simulink model "8Bit_Processor"  (R2019b)
settings: Solver=FixedStepDiscrete  StartTime=0.0  StopTime=10.0  RelTol=1e-3
libraries: hdlsllib x127, simulink_extras x9
(part 2 of 4)

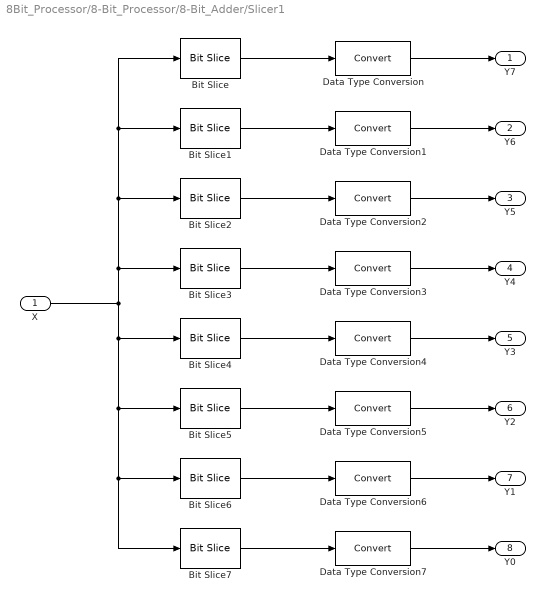
== system 8Bit_Processor/8-Bit_Processor/8-Bit_Adder/Slicer1 ==
  X : Inport  OutDataTypeStr=uint8  SampleTime=1
  Bit Slice : hdlsllib/Logic and Bit Operations/Bit Slice  lidx=7  ridx=7
      settings: SourceProductName=Simulink  SourceProductBaseCode=SL
  Bit Slice1 : hdlsllib/Logic and Bit Operations/Bit Slice  lidx=6  ridx=6
      settings: SourceProductName=Simulink  SourceProductBaseCode=SL
  Bit Slice2 : hdlsllib/Logic and Bit Operations/Bit Slice  lidx=5  ridx=5
      settings: SourceProductName=Simulink  SourceProductBaseCode=SL
  Bit Slice3 : hdlsllib/Logic and Bit Operations/Bit Slice  lidx=4  ridx=4
      settings: SourceProductName=Simulink  SourceProductBaseCode=SL
  Bit Slice4 : hdlsllib/Logic and Bit Operations/Bit Slice  lidx=3  ridx=3
      settings: SourceProductName=Simulink  SourceProductBaseCode=SL
  Bit Slice5 : hdlsllib/Logic and Bit Operations/Bit Slice  lidx=2  ridx=2
      settings: SourceProductName=Simulink  SourceProductBaseCode=SL
  Bit Slice6 : hdlsllib/Logic and Bit Operations/Bit Slice  lidx=1  ridx=1
      settings: SourceProductName=Simulink  SourceProductBaseCode=SL
  Bit Slice7 : hdlsllib/Logic and Bit Operations/Bit Slice  lidx=0  ridx=0
      settings: SourceProductName=Simulink  SourceProductBaseCode=SL
  Data Type Conversion{,1..7} (8 alike) : DataTypeConversion
  Y7 : Outport
  Y6 : Outport  Port=2
  Y5 : Outport  Port=3
  Y4 : Outport  Port=4
  Y3 : Outport  Port=5
  Y2 : Outport  Port=6
  Y1 : Outport  Port=7
  Y0 : Outport  Port=8
  wires:
  Bit Slice6/1 -> Data Type Conversion6/1
  X/1 -> Bit Slice3/1, Bit Slice2/1, Bit Slice1/1, Bit Slice/1, Bit Slice4/1, Bit Slice5/1, Bit Slice6/1, Bit Slice7/1
  Bit Slice/1 -> Data Type Conversion/1
  Bit Slice7/1 -> Data Type Conversion7/1
  Bit Slice4/1 -> Data Type Conversion4/1
  Bit Slice1/1 -> Data Type Conversion1/1
  Bit Slice3/1 -> Data Type Conversion3/1
  Data Type Conversion1/1 -> Y6/1
  Data Type Conversion7/1 -> Y0/1
  Data Type Conversion5/1 -> Y2/1
  Data Type Conversion3/1 -> Y4/1
  Data Type Conversion4/1 -> Y3/1
  Bit Slice2/1 -> Data Type Conversion2/1
  Bit Slice5/1 -> Data Type Conversion5/1
  Data Type Conversion6/1 -> Y1/1
  Data Type Conversion/1 -> Y7/1
  Data Type Conversion2/1 -> Y5/1

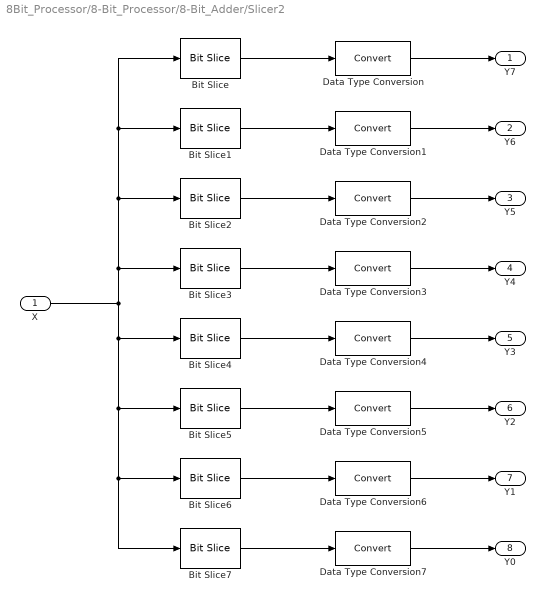
== system 8Bit_Processor/8-Bit_Processor/8-Bit_Adder/Slicer2 ==
  X : Inport  OutDataTypeStr=uint8  SampleTime=1
  Bit Slice : hdlsllib/Logic and Bit Operations/Bit Slice  lidx=7  ridx=7
      settings: SourceProductName=Simulink  SourceProductBaseCode=SL
  Bit Slice1 : hdlsllib/Logic and Bit Operations/Bit Slice  lidx=6  ridx=6
      settings: SourceProductName=Simulink  SourceProductBaseCode=SL
  Bit Slice2 : hdlsllib/Logic and Bit Operations/Bit Slice  lidx=5  ridx=5
      settings: SourceProductName=Simulink  SourceProductBaseCode=SL
  Bit Slice3 : hdlsllib/Logic and Bit Operations/Bit Slice  lidx=4  ridx=4
      settings: SourceProductName=Simulink  SourceProductBaseCode=SL
  Bit Slice4 : hdlsllib/Logic and Bit Operations/Bit Slice  lidx=3  ridx=3
      settings: SourceProductName=Simulink  SourceProductBaseCode=SL
  Bit Slice5 : hdlsllib/Logic and Bit Operations/Bit Slice  lidx=2  ridx=2
      settings: SourceProductName=Simulink  SourceProductBaseCode=SL
  Bit Slice6 : hdlsllib/Logic and Bit Operations/Bit Slice  lidx=1  ridx=1
      settings: SourceProductName=Simulink  SourceProductBaseCode=SL
  Bit Slice7 : hdlsllib/Logic and Bit Operations/Bit Slice  lidx=0  ridx=0
      settings: SourceProductName=Simulink  SourceProductBaseCode=SL
  Data Type Conversion{,1..7} (8 alike) : DataTypeConversion
  Y7 : Outport
  Y6 : Outport  Port=2
  Y5 : Outport  Port=3
  Y4 : Outport  Port=4
  Y3 : Outport  Port=5
  Y2 : Outport  Port=6
  Y1 : Outport  Port=7
  Y0 : Outport  Port=8
  wires:
  Bit Slice6/1 -> Data Type Conversion6/1
  X/1 -> Bit Slice3/1, Bit Slice2/1, Bit Slice1/1, Bit Slice/1, Bit Slice4/1, Bit Slice5/1, Bit Slice6/1, Bit Slice7/1
  Bit Slice/1 -> Data Type Conversion/1
  Bit Slice7/1 -> Data Type Conversion7/1
  Bit Slice4/1 -> Data Type Conversion4/1
  Bit Slice1/1 -> Data Type Conversion1/1
  Bit Slice3/1 -> Data Type Conversion3/1
  Data Type Conversion1/1 -> Y6/1
  Data Type Conversion7/1 -> Y0/1
  Data Type Conversion5/1 -> Y2/1
  Data Type Conversion3/1 -> Y4/1
  Data Type Conversion4/1 -> Y3/1
  Bit Slice2/1 -> Data Type Conversion2/1
  Bit Slice5/1 -> Data Type Conversion5/1
  Data Type Conversion6/1 -> Y1/1
  Data Type Conversion/1 -> Y7/1
  Data Type Conversion2/1 -> Y5/1

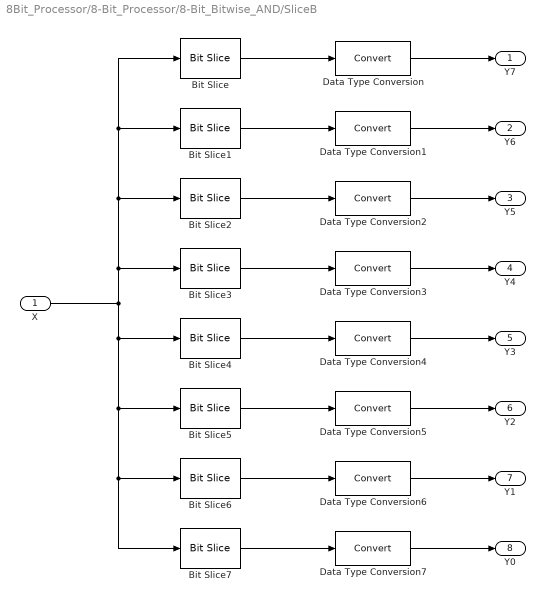
== system 8Bit_Processor/8-Bit_Processor/8-Bit_Bitwise_AND/SliceB ==
  X : Inport  OutDataTypeStr=uint8  SampleTime=1
  Bit Slice : hdlsllib/Logic and Bit Operations/Bit Slice  lidx=7  ridx=7
      settings: SourceProductName=Simulink  SourceProductBaseCode=SL
  Bit Slice1 : hdlsllib/Logic and Bit Operations/Bit Slice  lidx=6  ridx=6
      settings: SourceProductName=Simulink  SourceProductBaseCode=SL
  Bit Slice2 : hdlsllib/Logic and Bit Operations/Bit Slice  lidx=5  ridx=5
      settings: SourceProductName=Simulink  SourceProductBaseCode=SL
  Bit Slice3 : hdlsllib/Logic and Bit Operations/Bit Slice  lidx=4  ridx=4
      settings: SourceProductName=Simulink  SourceProductBaseCode=SL
  Bit Slice4 : hdlsllib/Logic and Bit Operations/Bit Slice  lidx=3  ridx=3
      settings: SourceProductName=Simulink  SourceProductBaseCode=SL
  Bit Slice5 : hdlsllib/Logic and Bit Operations/Bit Slice  lidx=2  ridx=2
      settings: SourceProductName=Simulink  SourceProductBaseCode=SL
  Bit Slice6 : hdlsllib/Logic and Bit Operations/Bit Slice  lidx=1  ridx=1
      settings: SourceProductName=Simulink  SourceProductBaseCode=SL
  Bit Slice7 : hdlsllib/Logic and Bit Operations/Bit Slice  lidx=0  ridx=0
      settings: SourceProductName=Simulink  SourceProductBaseCode=SL
  Data Type Conversion{,1..7} (8 alike) : DataTypeConversion
  Y7 : Outport
  Y6 : Outport  Port=2
  Y5 : Outport  Port=3
  Y4 : Outport  Port=4
  Y3 : Outport  Port=5
  Y2 : Outport  Port=6
  Y1 : Outport  Port=7
  Y0 : Outport  Port=8
  wires:
  Bit Slice6/1 -> Data Type Conversion6/1
  X/1 -> Bit Slice3/1, Bit Slice2/1, Bit Slice1/1, Bit Slice/1, Bit Slice4/1, Bit Slice5/1, Bit Slice6/1, Bit Slice7/1
  Bit Slice/1 -> Data Type Conversion/1
  Bit Slice7/1 -> Data Type Conversion7/1
  Bit Slice4/1 -> Data Type Conversion4/1
  Bit Slice1/1 -> Data Type Conversion1/1
  Bit Slice3/1 -> Data Type Conversion3/1
  Data Type Conversion1/1 -> Y6/1
  Data Type Conversion7/1 -> Y0/1
  Data Type Conversion5/1 -> Y2/1
  Data Type Conversion3/1 -> Y4/1
  Data Type Conversion4/1 -> Y3/1
  Bit Slice2/1 -> Data Type Conversion2/1
  Bit Slice5/1 -> Data Type Conversion5/1
  Data Type Conversion6/1 -> Y1/1
  Data Type Conversion/1 -> Y7/1
  Data Type Conversion2/1 -> Y5/1

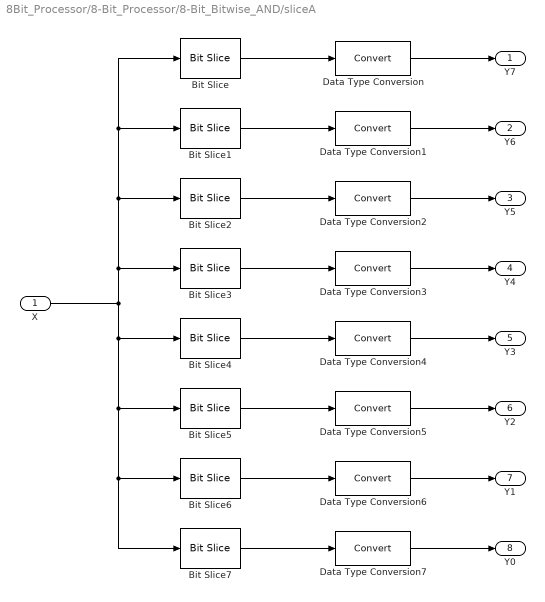
== system 8Bit_Processor/8-Bit_Processor/8-Bit_Bitwise_AND/sliceA ==
  X : Inport  OutDataTypeStr=uint8  SampleTime=1
  Bit Slice : hdlsllib/Logic and Bit Operations/Bit Slice  lidx=7  ridx=7
      settings: SourceProductName=Simulink  SourceProductBaseCode=SL
  Bit Slice1 : hdlsllib/Logic and Bit Operations/Bit Slice  lidx=6  ridx=6
      settings: SourceProductName=Simulink  SourceProductBaseCode=SL
  Bit Slice2 : hdlsllib/Logic and Bit Operations/Bit Slice  lidx=5  ridx=5
      settings: SourceProductName=Simulink  SourceProductBaseCode=SL
  Bit Slice3 : hdlsllib/Logic and Bit Operations/Bit Slice  lidx=4  ridx=4
      settings: SourceProductName=Simulink  SourceProductBaseCode=SL
  Bit Slice4 : hdlsllib/Logic and Bit Operations/Bit Slice  lidx=3  ridx=3
      settings: SourceProductName=Simulink  SourceProductBaseCode=SL
  Bit Slice5 : hdlsllib/Logic and Bit Operations/Bit Slice  lidx=2  ridx=2
      settings: SourceProductName=Simulink  SourceProductBaseCode=SL
  Bit Slice6 : hdlsllib/Logic and Bit Operations/Bit Slice  lidx=1  ridx=1
      settings: SourceProductName=Simulink  SourceProductBaseCode=SL
  Bit Slice7 : hdlsllib/Logic and Bit Operations/Bit Slice  lidx=0  ridx=0
      settings: SourceProductName=Simulink  SourceProductBaseCode=SL
  Data Type Conversion{,1..7} (8 alike) : DataTypeConversion
  Y7 : Outport
  Y6 : Outport  Port=2
  Y5 : Outport  Port=3
  Y4 : Outport  Port=4
  Y3 : Outport  Port=5
  Y2 : Outport  Port=6
  Y1 : Outport  Port=7
  Y0 : Outport  Port=8
  wires:
  Bit Slice6/1 -> Data Type Conversion6/1
  X/1 -> Bit Slice3/1, Bit Slice2/1, Bit Slice1/1, Bit Slice/1, Bit Slice4/1, Bit Slice5/1, Bit Slice6/1, Bit Slice7/1
  Bit Slice/1 -> Data Type Conversion/1
  Bit Slice7/1 -> Data Type Conversion7/1
  Bit Slice4/1 -> Data Type Conversion4/1
  Bit Slice1/1 -> Data Type Conversion1/1
  Bit Slice3/1 -> Data Type Conversion3/1
  Data Type Conversion1/1 -> Y6/1
  Data Type Conversion7/1 -> Y0/1
  Data Type Conversion5/1 -> Y2/1
  Data Type Conversion3/1 -> Y4/1
  Data Type Conversion4/1 -> Y3/1
  Bit Slice2/1 -> Data Type Conversion2/1
  Bit Slice5/1 -> Data Type Conversion5/1
  Data Type Conversion6/1 -> Y1/1
  Data Type Conversion/1 -> Y7/1
  Data Type Conversion2/1 -> Y5/1

== system 8Bit_Processor/8-Bit_Processor/8-Bit_Multiplier/Concat1 ==
  X0 : Inport  OutDataTypeStr=boolean  SampleTime=1
  X1 : Inport  Port=2  OutDataTypeStr=boolean  SampleTime=1
  X2 : Inport  Port=3  OutDataTypeStr=boolean  SampleTime=1
  X3 : Inport  Port=4  OutDataTypeStr=boolean  SampleTime=1
  X4 : Inport  Port=5  OutDataTypeStr=boolean  SampleTime=1
  X5 : Inport  Port=6  OutDataTypeStr=boolean  SampleTime=1
  X6 : Inport  Port=7  OutDataTypeStr=boolean  SampleTime=1
  X7 : Inport  Port=8  OutDataTypeStr=boolean  SampleTime=1
  Bit Concat : hdlsllib/Logic and Bit Operations/Bit Concat  numInputs=8
      settings: SourceProductName=Simulink
  Y : Outport
  wires:
  X6/1 -> Bit Concat/2
  X2/1 -> Bit Concat/6
  X7/1 -> Bit Concat/1
  X0/1 -> Bit Concat/8
  Bit Concat/1 -> Y/1
  X3/1 -> Bit Concat/5
  X1/1 -> Bit Concat/7
  X5/1 -> Bit Concat/3
  X4/1 -> Bit Concat/4

== system 8Bit_Processor/8-Bit_Processor/8-Bit_Multiplier/Full adder1 ==
  In1 : Inport  OutDataTypeStr=boolean
  In2 : Inport  Port=2  OutDataTypeStr=boolean
  In3 : Inport  Port=3  OutDataTypeStr=boolean
  Half adder1 : Subsystem
  Half adder2 : Subsystem
  Logical Operator1 : Logic  Operator=OR  AllPortsSameDT=off  OutDataTypeStr=boolean
  Out1 : Outport
  Out2 : Outport  Port=2
  wires:
  Logical Operator1/1 -> Out2/1
  In1/1 -> Half adder1/1(In1)
  Half adder2/1(Out1) -> Out1/1
  In2/1 -> Half adder1/2(In2)
  In3/1 -> Half adder2/2(In2)
  Half adder1/2(Out2) -> Logical Operator1/2
  Half adder1/1(Out1) -> Half adder2/1(In1)
  Half adder2/2(Out2) -> Logical Operator1/1

== system 8Bit_Processor/8-Bit_Processor/8-Bit_Multiplier/Full adder10 ==
  In1 : Inport  OutDataTypeStr=boolean
  In2 : Inport  Port=2  OutDataTypeStr=boolean
  In3 : Inport  Port=3  OutDataTypeStr=boolean
  Half adder1 : Subsystem
  Half adder2 : Subsystem
  Logical Operator1 : Logic  Operator=OR  AllPortsSameDT=off  OutDataTypeStr=boolean
  Out1 : Outport
  Out2 : Outport  Port=2
  wires:
  Logical Operator1/1 -> Out2/1
  In1/1 -> Half adder1/1(In1)
  Half adder2/1(Out1) -> Out1/1
  In2/1 -> Half adder1/2(In2)
  In3/1 -> Half adder2/2(In2)
  Half adder1/2(Out2) -> Logical Operator1/2
  Half adder1/1(Out1) -> Half adder2/1(In1)
  Half adder2/2(Out2) -> Logical Operator1/1

== system 8Bit_Processor/8-Bit_Processor/8-Bit_Multiplier/Full adder11 ==
  In1 : Inport  OutDataTypeStr=boolean
  In2 : Inport  Port=2  OutDataTypeStr=boolean
  In3 : Inport  Port=3  OutDataTypeStr=boolean
  Half adder1 : Subsystem
  Half adder2 : Subsystem
  Logical Operator1 : Logic  Operator=OR  AllPortsSameDT=off  OutDataTypeStr=boolean
  Out1 : Outport
  Out2 : Outport  Port=2
  wires:
  Logical Operator1/1 -> Out2/1
  In1/1 -> Half adder1/1(In1)
  Half adder2/1(Out1) -> Out1/1
  In2/1 -> Half adder1/2(In2)
  In3/1 -> Half adder2/2(In2)
  Half adder1/2(Out2) -> Logical Operator1/2
  Half adder1/1(Out1) -> Half adder2/1(In1)
  Half adder2/2(Out2) -> Logical Operator1/1

== system 8Bit_Processor/8-Bit_Processor/8-Bit_Multiplier/Full adder12 ==
  In1 : Inport  OutDataTypeStr=boolean
  In2 : Inport  Port=2  OutDataTypeStr=boolean
  In3 : Inport  Port=3  OutDataTypeStr=boolean
  Half adder1 : Subsystem
  Half adder2 : Subsystem
  Logical Operator1 : Logic  Operator=OR  AllPortsSameDT=off  OutDataTypeStr=boolean
  Out1 : Outport
  Out2 : Outport  Port=2
  wires:
  Logical Operator1/1 -> Out2/1
  In1/1 -> Half adder1/1(In1)
  Half adder2/1(Out1) -> Out1/1
  In2/1 -> Half adder1/2(In2)
  In3/1 -> Half adder2/2(In2)
  Half adder1/2(Out2) -> Logical Operator1/2
  Half adder1/1(Out1) -> Half adder2/1(In1)
  Half adder2/2(Out2) -> Logical Operator1/1

== system 8Bit_Processor/8-Bit_Processor/8-Bit_Multiplier/Full adder13 ==
  In1 : Inport  OutDataTypeStr=boolean
  In2 : Inport  Port=2  OutDataTypeStr=boolean
  In3 : Inport  Port=3  OutDataTypeStr=boolean
  Half adder1 : Subsystem
  Half adder2 : Subsystem
  Logical Operator1 : Logic  Operator=OR  AllPortsSameDT=off  OutDataTypeStr=boolean
  Out1 : Outport
  Out2 : Outport  Port=2
  wires:
  Logical Operator1/1 -> Out2/1
  In1/1 -> Half adder1/1(In1)
  Half adder2/1(Out1) -> Out1/1
  In2/1 -> Half adder1/2(In2)
  In3/1 -> Half adder2/2(In2)
  Half adder1/2(Out2) -> Logical Operator1/2
  Half adder1/1(Out1) -> Half adder2/1(In1)
  Half adder2/2(Out2) -> Logical Operator1/1

== system 8Bit_Processor/8-Bit_Processor/8-Bit_Multiplier/Full adder14 ==
  In1 : Inport  OutDataTypeStr=boolean
  In2 : Inport  Port=2  OutDataTypeStr=boolean
  In3 : Inport  Port=3  OutDataTypeStr=boolean
  Half adder1 : Subsystem
  Half adder2 : Subsystem
  Logical Operator1 : Logic  Operator=OR  AllPortsSameDT=off  OutDataTypeStr=boolean
  Out1 : Outport
  Out2 : Outport  Port=2
  wires:
  Logical Operator1/1 -> Out2/1
  In1/1 -> Half adder1/1(In1)
  Half adder2/1(Out1) -> Out1/1
  In2/1 -> Half adder1/2(In2)
  In3/1 -> Half adder2/2(In2)
  Half adder1/2(Out2) -> Logical Operator1/2
  Half adder1/1(Out1) -> Half adder2/1(In1)
  Half adder2/2(Out2) -> Logical Operator1/1

== system 8Bit_Processor/8-Bit_Processor/8-Bit_Multiplier/Full adder15 ==
  In1 : Inport  OutDataTypeStr=boolean
  In2 : Inport  Port=2  OutDataTypeStr=boolean
  In3 : Inport  Port=3  OutDataTypeStr=boolean
  Half adder1 : Subsystem
  Half adder2 : Subsystem
  Logical Operator1 : Logic  Operator=OR  AllPortsSameDT=off  OutDataTypeStr=boolean
  Out1 : Outport
  Out2 : Outport  Port=2
  wires:
  Logical Operator1/1 -> Out2/1
  In1/1 -> Half adder1/1(In1)
  Half adder2/1(Out1) -> Out1/1
  In2/1 -> Half adder1/2(In2)
  In3/1 -> Half adder2/2(In2)
  Half adder1/2(Out2) -> Logical Operator1/2
  Half adder1/1(Out1) -> Half adder2/1(In1)
  Half adder2/2(Out2) -> Logical Operator1/1

== system 8Bit_Processor/8-Bit_Processor/8-Bit_Multiplier/Full adder16 ==
  In1 : Inport  OutDataTypeStr=boolean
  In2 : Inport  Port=2  OutDataTypeStr=boolean
  In3 : Inport  Port=3  OutDataTypeStr=boolean
  Half adder1 : Subsystem
  Half adder2 : Subsystem
  Logical Operator1 : Logic  Operator=OR  AllPortsSameDT=off  OutDataTypeStr=boolean
  Out1 : Outport
  Out2 : Outport  Port=2
  wires:
  Logical Operator1/1 -> Out2/1
  In1/1 -> Half adder1/1(In1)
  Half adder2/1(Out1) -> Out1/1
  In2/1 -> Half adder1/2(In2)
  In3/1 -> Half adder2/2(In2)
  Half adder1/2(Out2) -> Logical Operator1/2
  Half adder1/1(Out1) -> Half adder2/1(In1)
  Half adder2/2(Out2) -> Logical Operator1/1

== system 8Bit_Processor/8-Bit_Processor/8-Bit_Multiplier/Full adder17 ==
  In1 : Inport  OutDataTypeStr=boolean
  In2 : Inport  Port=2  OutDataTypeStr=boolean
  In3 : Inport  Port=3  OutDataTypeStr=boolean
  Half adder1 : Subsystem
  Half adder2 : Subsystem
  Logical Operator1 : Logic  Operator=OR  AllPortsSameDT=off  OutDataTypeStr=boolean
  Out1 : Outport
  Out2 : Outport  Port=2
  wires:
  Logical Operator1/1 -> Out2/1
  In1/1 -> Half adder1/1(In1)
  Half adder2/1(Out1) -> Out1/1
  In2/1 -> Half adder1/2(In2)
  In3/1 -> Half adder2/2(In2)
  Half adder1/2(Out2) -> Logical Operator1/2
  Half adder1/1(Out1) -> Half adder2/1(In1)
  Half adder2/2(Out2) -> Logical Operator1/1

== system 8Bit_Processor/8-Bit_Processor/8-Bit_Multiplier/Full adder18 ==
  In1 : Inport  OutDataTypeStr=boolean
  In2 : Inport  Port=2  OutDataTypeStr=boolean
  In3 : Inport  Port=3  OutDataTypeStr=boolean
  Half adder1 : Subsystem
  Half adder2 : Subsystem
  Logical Operator1 : Logic  Operator=OR  AllPortsSameDT=off  OutDataTypeStr=boolean
  Out1 : Outport
  Out2 : Outport  Port=2
  wires:
  Logical Operator1/1 -> Out2/1
  In1/1 -> Half adder1/1(In1)
  Half adder2/1(Out1) -> Out1/1
  In2/1 -> Half adder1/2(In2)
  In3/1 -> Half adder2/2(In2)
  Half adder1/2(Out2) -> Logical Operator1/2
  Half adder1/1(Out1) -> Half adder2/1(In1)
  Half adder2/2(Out2) -> Logical Operator1/1

== system 8Bit_Processor/8-Bit_Processor/8-Bit_Multiplier/Full adder19 ==
  In1 : Inport  OutDataTypeStr=boolean
  In2 : Inport  Port=2  OutDataTypeStr=boolean
  In3 : Inport  Port=3  OutDataTypeStr=boolean
  Half adder1 : Subsystem
  Half adder2 : Subsystem
  Logical Operator1 : Logic  Operator=OR  AllPortsSameDT=off  OutDataTypeStr=boolean
  Out1 : Outport
  Out2 : Outport  Port=2
  wires:
  Logical Operator1/1 -> Out2/1
  In1/1 -> Half adder1/1(In1)
  Half adder2/1(Out1) -> Out1/1
  In2/1 -> Half adder1/2(In2)
  In3/1 -> Half adder2/2(In2)
  Half adder1/2(Out2) -> Logical Operator1/2
  Half adder1/1(Out1) -> Half adder2/1(In1)
  Half adder2/2(Out2) -> Logical Operator1/1

== system 8Bit_Processor/8-Bit_Processor/8-Bit_Multiplier/Full adder2 ==
  In1 : Inport  OutDataTypeStr=boolean
  In2 : Inport  Port=2  OutDataTypeStr=boolean
  In3 : Inport  Port=3  OutDataTypeStr=boolean
  Half adder1 : Subsystem
  Half adder2 : Subsystem
  Logical Operator1 : Logic  Operator=OR  AllPortsSameDT=off  OutDataTypeStr=boolean
  Out1 : Outport
  Out2 : Outport  Port=2
  wires:
  Logical Operator1/1 -> Out2/1
  In1/1 -> Half adder1/1(In1)
  Half adder2/1(Out1) -> Out1/1
  In2/1 -> Half adder1/2(In2)
  In3/1 -> Half adder2/2(In2)
  Half adder1/2(Out2) -> Logical Operator1/2
  Half adder1/1(Out1) -> Half adder2/1(In1)
  Half adder2/2(Out2) -> Logical Operator1/1

== system 8Bit_Processor/8-Bit_Processor/8-Bit_Multiplier/Full adder20 ==
  In1 : Inport  OutDataTypeStr=boolean
  In2 : Inport  Port=2  OutDataTypeStr=boolean
  In3 : Inport  Port=3  OutDataTypeStr=boolean
  Half adder1 : Subsystem
  Half adder2 : Subsystem
  Logical Operator1 : Logic  Operator=OR  AllPortsSameDT=off  OutDataTypeStr=boolean
  Out1 : Outport
  Out2 : Outport  Port=2
  wires:
  Logical Operator1/1 -> Out2/1
  In1/1 -> Half adder1/1(In1)
  Half adder2/1(Out1) -> Out1/1
  In2/1 -> Half adder1/2(In2)
  In3/1 -> Half adder2/2(In2)
  Half adder1/2(Out2) -> Logical Operator1/2
  Half adder1/1(Out1) -> Half adder2/1(In1)
  Half adder2/2(Out2) -> Logical Operator1/1

== system 8Bit_Processor/8-Bit_Processor/8-Bit_Multiplier/Full adder21 ==
  In1 : Inport  OutDataTypeStr=boolean
  In2 : Inport  Port=2  OutDataTypeStr=boolean
  In3 : Inport  Port=3  OutDataTypeStr=boolean
  Half adder1 : Subsystem
  Half adder2 : Subsystem
  Logical Operator1 : Logic  Operator=OR  AllPortsSameDT=off  OutDataTypeStr=boolean
  Out1 : Outport
  Out2 : Outport  Port=2
  wires:
  Logical Operator1/1 -> Out2/1
  In1/1 -> Half adder1/1(In1)
  Half adder2/1(Out1) -> Out1/1
  In2/1 -> Half adder1/2(In2)
  In3/1 -> Half adder2/2(In2)
  Half adder1/2(Out2) -> Logical Operator1/2
  Half adder1/1(Out1) -> Half adder2/1(In1)
  Half adder2/2(Out2) -> Logical Operator1/1

== system 8Bit_Processor/8-Bit_Processor/8-Bit_Multiplier/Full adder22 ==
  In1 : Inport  OutDataTypeStr=boolean
  In2 : Inport  Port=2  OutDataTypeStr=boolean
  In3 : Inport  Port=3  OutDataTypeStr=boolean
  Half adder1 : Subsystem
  Half adder2 : Subsystem
  Logical Operator1 : Logic  Operator=OR  AllPortsSameDT=off  OutDataTypeStr=boolean
  Out1 : Outport
  Out2 : Outport  Port=2
  wires:
  Logical Operator1/1 -> Out2/1
  In1/1 -> Half adder1/1(In1)
  Half adder2/1(Out1) -> Out1/1
  In2/1 -> Half adder1/2(In2)
  In3/1 -> Half adder2/2(In2)
  Half adder1/2(Out2) -> Logical Operator1/2
  Half adder1/1(Out1) -> Half adder2/1(In1)
  Half adder2/2(Out2) -> Logical Operator1/1

== system 8Bit_Processor/8-Bit_Processor/8-Bit_Multiplier/Full adder23 ==
  In1 : Inport  OutDataTypeStr=boolean
  In2 : Inport  Port=2  OutDataTypeStr=boolean
  In3 : Inport  Port=3  OutDataTypeStr=boolean
  Half adder1 : Subsystem
  Half adder2 : Subsystem
  Logical Operator1 : Logic  Operator=OR  AllPortsSameDT=off  OutDataTypeStr=boolean
  Out1 : Outport
  Out2 : Outport  Port=2
  wires:
  Logical Operator1/1 -> Out2/1
  In1/1 -> Half adder1/1(In1)
  Half adder2/1(Out1) -> Out1/1
  In2/1 -> Half adder1/2(In2)
  In3/1 -> Half adder2/2(In2)
  Half adder1/2(Out2) -> Logical Operator1/2
  Half adder1/1(Out1) -> Half adder2/1(In1)
  Half adder2/2(Out2) -> Logical Operator1/1

== system 8Bit_Processor/8-Bit_Processor/8-Bit_Multiplier/Full adder24 ==
  In1 : Inport  OutDataTypeStr=boolean
  In2 : Inport  Port=2  OutDataTypeStr=boolean
  In3 : Inport  Port=3  OutDataTypeStr=boolean
  Half adder1 : Subsystem
  Half adder2 : Subsystem
  Logical Operator1 : Logic  Operator=OR  AllPortsSameDT=off  OutDataTypeStr=boolean
  Out1 : Outport
  Out2 : Outport  Port=2
  wires:
  Logical Operator1/1 -> Out2/1
  In1/1 -> Half adder1/1(In1)
  Half adder2/1(Out1) -> Out1/1
  In2/1 -> Half adder1/2(In2)
  In3/1 -> Half adder2/2(In2)
  Half adder1/2(Out2) -> Logical Operator1/2
  Half adder1/1(Out1) -> Half adder2/1(In1)
  Half adder2/2(Out2) -> Logical Operator1/1

== system 8Bit_Processor/8-Bit_Processor/8-Bit_Multiplier/Full adder25 ==
  In1 : Inport  OutDataTypeStr=boolean
  In2 : Inport  Port=2  OutDataTypeStr=boolean
  In3 : Inport  Port=3  OutDataTypeStr=boolean
  Half adder1 : Subsystem
  Half adder2 : Subsystem
  Logical Operator1 : Logic  Operator=OR  AllPortsSameDT=off  OutDataTypeStr=boolean
  Out1 : Outport
  Out2 : Outport  Port=2
  wires:
  Logical Operator1/1 -> Out2/1
  In1/1 -> Half adder1/1(In1)
  Half adder2/1(Out1) -> Out1/1
  In2/1 -> Half adder1/2(In2)
  In3/1 -> Half adder2/2(In2)
  Half adder1/2(Out2) -> Logical Operator1/2
  Half adder1/1(Out1) -> Half adder2/1(In1)
  Half adder2/2(Out2) -> Logical Operator1/1

== system 8Bit_Processor/8-Bit_Processor/8-Bit_Multiplier/Full adder26 ==
  In1 : Inport  OutDataTypeStr=boolean
  In2 : Inport  Port=2  OutDataTypeStr=boolean
  In3 : Inport  Port=3  OutDataTypeStr=boolean
  Half adder1 : Subsystem
  Half adder2 : Subsystem
  Logical Operator1 : Logic  Operator=OR  AllPortsSameDT=off  OutDataTypeStr=boolean
  Out1 : Outport
  Out2 : Outport  Port=2
  wires:
  Logical Operator1/1 -> Out2/1
  In1/1 -> Half adder1/1(In1)
  Half adder2/1(Out1) -> Out1/1
  In2/1 -> Half adder1/2(In2)
  In3/1 -> Half adder2/2(In2)
  Half adder1/2(Out2) -> Logical Operator1/2
  Half adder1/1(Out1) -> Half adder2/1(In1)
  Half adder2/2(Out2) -> Logical Operator1/1

== system 8Bit_Processor/8-Bit_Processor/8-Bit_Multiplier/Full adder27 ==
  In1 : Inport  OutDataTypeStr=boolean
  In2 : Inport  Port=2  OutDataTypeStr=boolean
  In3 : Inport  Port=3  OutDataTypeStr=boolean
  Half adder1 : Subsystem
  Half adder2 : Subsystem
  Logical Operator1 : Logic  Operator=OR  AllPortsSameDT=off  OutDataTypeStr=boolean
  Out1 : Outport
  Out2 : Outport  Port=2
  wires:
  Logical Operator1/1 -> Out2/1
  In1/1 -> Half adder1/1(In1)
  Half adder2/1(Out1) -> Out1/1
  In2/1 -> Half adder1/2(In2)
  In3/1 -> Half adder2/2(In2)
  Half adder1/2(Out2) -> Logical Operator1/2
  Half adder1/1(Out1) -> Half adder2/1(In1)
  Half adder2/2(Out2) -> Logical Operator1/1

== system 8Bit_Processor/8-Bit_Processor/8-Bit_Multiplier/Full adder28 ==
  In1 : Inport  OutDataTypeStr=boolean
  In2 : Inport  Port=2  OutDataTypeStr=boolean
  In3 : Inport  Port=3  OutDataTypeStr=boolean
  Half adder1 : Subsystem
  Half adder2 : Subsystem
  Logical Operator1 : Logic  Operator=OR  AllPortsSameDT=off  OutDataTypeStr=boolean
  Out1 : Outport
  Out2 : Outport  Port=2
  wires:
  Logical Operator1/1 -> Out2/1
  In1/1 -> Half adder1/1(In1)
  Half adder2/1(Out1) -> Out1/1
  In2/1 -> Half adder1/2(In2)
  In3/1 -> Half adder2/2(In2)
  Half adder1/2(Out2) -> Logical Operator1/2
  Half adder1/1(Out1) -> Half adder2/1(In1)
  Half adder2/2(Out2) -> Logical Operator1/1

== system 8Bit_Processor/8-Bit_Processor/8-Bit_Multiplier/Full adder29 ==
  In1 : Inport  OutDataTypeStr=boolean
  In2 : Inport  Port=2  OutDataTypeStr=boolean
  In3 : Inport  Port=3  OutDataTypeStr=boolean
  Half adder1 : Subsystem
  Half adder2 : Subsystem
  Logical Operator1 : Logic  Operator=OR  AllPortsSameDT=off  OutDataTypeStr=boolean
  Out1 : Outport
  Out2 : Outport  Port=2
  wires:
  Logical Operator1/1 -> Out2/1
  In1/1 -> Half adder1/1(In1)
  Half adder2/1(Out1) -> Out1/1
  In2/1 -> Half adder1/2(In2)
  In3/1 -> Half adder2/2(In2)
  Half adder1/2(Out2) -> Logical Operator1/2
  Half adder1/1(Out1) -> Half adder2/1(In1)
  Half adder2/2(Out2) -> Logical Operator1/1

== system 8Bit_Processor/8-Bit_Processor/8-Bit_Multiplier/Full adder3 ==
  In1 : Inport  OutDataTypeStr=boolean
  In2 : Inport  Port=2  OutDataTypeStr=boolean
  In3 : Inport  Port=3  OutDataTypeStr=boolean
  Half adder1 : Subsystem
  Half adder2 : Subsystem
  Logical Operator1 : Logic  Operator=OR  AllPortsSameDT=off  OutDataTypeStr=boolean
  Out1 : Outport
  Out2 : Outport  Port=2
  wires:
  Logical Operator1/1 -> Out2/1
  In1/1 -> Half adder1/1(In1)
  Half adder2/1(Out1) -> Out1/1
  In2/1 -> Half adder1/2(In2)
  In3/1 -> Half adder2/2(In2)
  Half adder1/2(Out2) -> Logical Operator1/2
  Half adder1/1(Out1) -> Half adder2/1(In1)
  Half adder2/2(Out2) -> Logical Operator1/1

== system 8Bit_Processor/8-Bit_Processor/8-Bit_Multiplier/Full adder30 ==
  In1 : Inport  OutDataTypeStr=boolean
  In2 : Inport  Port=2  OutDataTypeStr=boolean
  In3 : Inport  Port=3  OutDataTypeStr=boolean
  Half adder1 : Subsystem
  Half adder2 : Subsystem
  Logical Operator1 : Logic  Operator=OR  AllPortsSameDT=off  OutDataTypeStr=boolean
  Out1 : Outport
  Out2 : Outport  Port=2
  wires:
  Logical Operator1/1 -> Out2/1
  In1/1 -> Half adder1/1(In1)
  Half adder2/1(Out1) -> Out1/1
  In2/1 -> Half adder1/2(In2)
  In3/1 -> Half adder2/2(In2)
  Half adder1/2(Out2) -> Logical Operator1/2
  Half adder1/1(Out1) -> Half adder2/1(In1)
  Half adder2/2(Out2) -> Logical Operator1/1

== system 8Bit_Processor/8-Bit_Processor/8-Bit_Multiplier/Full adder31 ==
  In1 : Inport  OutDataTypeStr=boolean
  In2 : Inport  Port=2  OutDataTypeStr=boolean
  In3 : Inport  Port=3  OutDataTypeStr=boolean
  Half adder1 : Subsystem
  Half adder2 : Subsystem
  Logical Operator1 : Logic  Operator=OR  AllPortsSameDT=off  OutDataTypeStr=boolean
  Out1 : Outport
  Out2 : Outport  Port=2
  wires:
  Logical Operator1/1 -> Out2/1
  In1/1 -> Half adder1/1(In1)
  Half adder2/1(Out1) -> Out1/1
  In2/1 -> Half adder1/2(In2)
  In3/1 -> Half adder2/2(In2)
  Half adder1/2(Out2) -> Logical Operator1/2
  Half adder1/1(Out1) -> Half adder2/1(In1)
  Half adder2/2(Out2) -> Logical Operator1/1

== system 8Bit_Processor/8-Bit_Processor/8-Bit_Multiplier/Full adder32 ==
  In1 : Inport  OutDataTypeStr=boolean
  In2 : Inport  Port=2  OutDataTypeStr=boolean
  In3 : Inport  Port=3  OutDataTypeStr=boolean
  Half adder1 : Subsystem
  Half adder2 : Subsystem
  Logical Operator1 : Logic  Operator=OR  AllPortsSameDT=off  OutDataTypeStr=boolean
  Out1 : Outport
  Out2 : Outport  Port=2
  wires:
  Logical Operator1/1 -> Out2/1
  In1/1 -> Half adder1/1(In1)
  Half adder2/1(Out1) -> Out1/1
  In2/1 -> Half adder1/2(In2)
  In3/1 -> Half adder2/2(In2)
  Half adder1/2(Out2) -> Logical Operator1/2
  Half adder1/1(Out1) -> Half adder2/1(In1)
  Half adder2/2(Out2) -> Logical Operator1/1

== system 8Bit_Processor/8-Bit_Processor/8-Bit_Multiplier/Full adder33 ==
  In1 : Inport  OutDataTypeStr=boolean
  In2 : Inport  Port=2  OutDataTypeStr=boolean
  In3 : Inport  Port=3  OutDataTypeStr=boolean
  Half adder1 : Subsystem
  Half adder2 : Subsystem
  Logical Operator1 : Logic  Operator=OR  AllPortsSameDT=off  OutDataTypeStr=boolean
  Out1 : Outport
  Out2 : Outport  Port=2
  wires:
  Logical Operator1/1 -> Out2/1
  In1/1 -> Half adder1/1(In1)
  Half adder2/1(Out1) -> Out1/1
  In2/1 -> Half adder1/2(In2)
  In3/1 -> Half adder2/2(In2)
  Half adder1/2(Out2) -> Logical Operator1/2
  Half adder1/1(Out1) -> Half adder2/1(In1)
  Half adder2/2(Out2) -> Logical Operator1/1

== system 8Bit_Processor/8-Bit_Processor/8-Bit_Multiplier/Full adder34 ==
  In1 : Inport  OutDataTypeStr=boolean
  In2 : Inport  Port=2  OutDataTypeStr=boolean
  In3 : Inport  Port=3  OutDataTypeStr=boolean
  Half adder1 : Subsystem
  Half adder2 : Subsystem
  Logical Operator1 : Logic  Operator=OR  AllPortsSameDT=off  OutDataTypeStr=boolean
  Out1 : Outport
  Out2 : Outport  Port=2
  wires:
  Logical Operator1/1 -> Out2/1
  In1/1 -> Half adder1/1(In1)
  Half adder2/1(Out1) -> Out1/1
  In2/1 -> Half adder1/2(In2)
  In3/1 -> Half adder2/2(In2)
  Half adder1/2(Out2) -> Logical Operator1/2
  Half adder1/1(Out1) -> Half adder2/1(In1)
  Half adder2/2(Out2) -> Logical Operator1/1

== system 8Bit_Processor/8-Bit_Processor/8-Bit_Multiplier/Full adder35 ==
  In1 : Inport  OutDataTypeStr=boolean
  In2 : Inport  Port=2  OutDataTypeStr=boolean
  In3 : Inport  Port=3  OutDataTypeStr=boolean
  Half adder1 : Subsystem
  Half adder2 : Subsystem
  Logical Operator1 : Logic  Operator=OR  AllPortsSameDT=off  OutDataTypeStr=boolean
  Out1 : Outport
  Out2 : Outport  Port=2
  wires:
  Logical Operator1/1 -> Out2/1
  In1/1 -> Half adder1/1(In1)
  Half adder2/1(Out1) -> Out1/1
  In2/1 -> Half adder1/2(In2)
  In3/1 -> Half adder2/2(In2)
  Half adder1/2(Out2) -> Logical Operator1/2
  Half adder1/1(Out1) -> Half adder2/1(In1)
  Half adder2/2(Out2) -> Logical Operator1/1

== system 8Bit_Processor/8-Bit_Processor/8-Bit_Multiplier/Full adder36 ==
  In1 : Inport  OutDataTypeStr=boolean
  In2 : Inport  Port=2  OutDataTypeStr=boolean
  In3 : Inport  Port=3  OutDataTypeStr=boolean
  Half adder1 : Subsystem
  Half adder2 : Subsystem
  Logical Operator1 : Logic  Operator=OR  AllPortsSameDT=off  OutDataTypeStr=boolean
  Out1 : Outport
  Out2 : Outport  Port=2
  wires:
  Logical Operator1/1 -> Out2/1
  In1/1 -> Half adder1/1(In1)
  Half adder2/1(Out1) -> Out1/1
  In2/1 -> Half adder1/2(In2)
  In3/1 -> Half adder2/2(In2)
  Half adder1/2(Out2) -> Logical Operator1/2
  Half adder1/1(Out1) -> Half adder2/1(In1)
  Half adder2/2(Out2) -> Logical Operator1/1

== system 8Bit_Processor/8-Bit_Processor/8-Bit_Multiplier/Full adder37 ==
  In1 : Inport  OutDataTypeStr=boolean
  In2 : Inport  Port=2  OutDataTypeStr=boolean
  In3 : Inport  Port=3  OutDataTypeStr=boolean
  Half adder1 : Subsystem
  Half adder2 : Subsystem
  Logical Operator1 : Logic  Operator=OR  AllPortsSameDT=off  OutDataTypeStr=boolean
  Out1 : Outport
  Out2 : Outport  Port=2
  wires:
  Logical Operator1/1 -> Out2/1
  In1/1 -> Half adder1/1(In1)
  Half adder2/1(Out1) -> Out1/1
  In2/1 -> Half adder1/2(In2)
  In3/1 -> Half adder2/2(In2)
  Half adder1/2(Out2) -> Logical Operator1/2
  Half adder1/1(Out1) -> Half adder2/1(In1)
  Half adder2/2(Out2) -> Logical Operator1/1

== system 8Bit_Processor/8-Bit_Processor/8-Bit_Multiplier/Full adder38 ==
  In1 : Inport  OutDataTypeStr=boolean
  In2 : Inport  Port=2  OutDataTypeStr=boolean
  In3 : Inport  Port=3  OutDataTypeStr=boolean
  Half adder1 : Subsystem
  Half adder2 : Subsystem
  Logical Operator1 : Logic  Operator=OR  AllPortsSameDT=off  OutDataTypeStr=boolean
  Out1 : Outport
  Out2 : Outport  Port=2
  wires:
  Logical Operator1/1 -> Out2/1
  In1/1 -> Half adder1/1(In1)
  Half adder2/1(Out1) -> Out1/1
  In2/1 -> Half adder1/2(In2)
  In3/1 -> Half adder2/2(In2)
  Half adder1/2(Out2) -> Logical Operator1/2
  Half adder1/1(Out1) -> Half adder2/1(In1)
  Half adder2/2(Out2) -> Logical Operator1/1

== system 8Bit_Processor/8-Bit_Processor/8-Bit_Multiplier/Full adder39 ==
  In1 : Inport  OutDataTypeStr=boolean
  In2 : Inport  Port=2  OutDataTypeStr=boolean
  In3 : Inport  Port=3  OutDataTypeStr=boolean
  Half adder1 : Subsystem
  Half adder2 : Subsystem
  Logical Operator1 : Logic  Operator=OR  AllPortsSameDT=off  OutDataTypeStr=boolean
  Out1 : Outport
  Out2 : Outport  Port=2
  wires:
  Logical Operator1/1 -> Out2/1
  In1/1 -> Half adder1/1(In1)
  Half adder2/1(Out1) -> Out1/1
  In2/1 -> Half adder1/2(In2)
  In3/1 -> Half adder2/2(In2)
  Half adder1/2(Out2) -> Logical Operator1/2
  Half adder1/1(Out1) -> Half adder2/1(In1)
  Half adder2/2(Out2) -> Logical Operator1/1

== system 8Bit_Processor/8-Bit_Processor/8-Bit_Multiplier/Full adder4 ==
  In1 : Inport  OutDataTypeStr=boolean
  In2 : Inport  Port=2  OutDataTypeStr=boolean
  In3 : Inport  Port=3  OutDataTypeStr=boolean
  Half adder1 : Subsystem
  Half adder2 : Subsystem
  Logical Operator1 : Logic  Operator=OR  AllPortsSameDT=off  OutDataTypeStr=boolean
  Out1 : Outport
  Out2 : Outport  Port=2
  wires:
  Logical Operator1/1 -> Out2/1
  In1/1 -> Half adder1/1(In1)
  Half adder2/1(Out1) -> Out1/1
  In2/1 -> Half adder1/2(In2)
  In3/1 -> Half adder2/2(In2)
  Half adder1/2(Out2) -> Logical Operator1/2
  Half adder1/1(Out1) -> Half adder2/1(In1)
  Half adder2/2(Out2) -> Logical Operator1/1

== system 8Bit_Processor/8-Bit_Processor/8-Bit_Multiplier/Full adder40 ==
  In1 : Inport  OutDataTypeStr=boolean
  In2 : Inport  Port=2  OutDataTypeStr=boolean
  In3 : Inport  Port=3  OutDataTypeStr=boolean
  Half adder1 : Subsystem
  Half adder2 : Subsystem
  Logical Operator1 : Logic  Operator=OR  AllPortsSameDT=off  OutDataTypeStr=boolean
  Out1 : Outport
  Out2 : Outport  Port=2
  wires:
  Logical Operator1/1 -> Out2/1
  In1/1 -> Half adder1/1(In1)
  Half adder2/1(Out1) -> Out1/1
  In2/1 -> Half adder1/2(In2)
  In3/1 -> Half adder2/2(In2)
  Half adder1/2(Out2) -> Logical Operator1/2
  Half adder1/1(Out1) -> Half adder2/1(In1)
  Half adder2/2(Out2) -> Logical Operator1/1

== system 8Bit_Processor/8-Bit_Processor/8-Bit_Multiplier/Full adder41 ==
  In1 : Inport  OutDataTypeStr=boolean
  In2 : Inport  Port=2  OutDataTypeStr=boolean
  In3 : Inport  Port=3  OutDataTypeStr=boolean
  Half adder1 : Subsystem
  Half adder2 : Subsystem
  Logical Operator1 : Logic  Operator=OR  AllPortsSameDT=off  OutDataTypeStr=boolean
  Out1 : Outport
  Out2 : Outport  Port=2
  wires:
  Logical Operator1/1 -> Out2/1
  In1/1 -> Half adder1/1(In1)
  Half adder2/1(Out1) -> Out1/1
  In2/1 -> Half adder1/2(In2)
  In3/1 -> Half adder2/2(In2)
  Half adder1/2(Out2) -> Logical Operator1/2
  Half adder1/1(Out1) -> Half adder2/1(In1)
  Half adder2/2(Out2) -> Logical Operator1/1

== system 8Bit_Processor/8-Bit_Processor/8-Bit_Multiplier/Full adder42 ==
  In1 : Inport  OutDataTypeStr=boolean
  In2 : Inport  Port=2  OutDataTypeStr=boolean
  In3 : Inport  Port=3  OutDataTypeStr=boolean
  Half adder1 : Subsystem
  Half adder2 : Subsystem
  Logical Operator1 : Logic  Operator=OR  AllPortsSameDT=off  OutDataTypeStr=boolean
  Out1 : Outport
  Out2 : Outport  Port=2
  wires:
  Logical Operator1/1 -> Out2/1
  In1/1 -> Half adder1/1(In1)
  Half adder2/1(Out1) -> Out1/1
  In2/1 -> Half adder1/2(In2)
  In3/1 -> Half adder2/2(In2)
  Half adder1/2(Out2) -> Logical Operator1/2
  Half adder1/1(Out1) -> Half adder2/1(In1)
  Half adder2/2(Out2) -> Logical Operator1/1

== system 8Bit_Processor/8-Bit_Processor/8-Bit_Multiplier/Full adder43 ==
  In1 : Inport  OutDataTypeStr=boolean
  In2 : Inport  Port=2  OutDataTypeStr=boolean
  In3 : Inport  Port=3  OutDataTypeStr=boolean
  Half adder1 : Subsystem
  Half adder2 : Subsystem
  Logical Operator1 : Logic  Operator=OR  AllPortsSameDT=off  OutDataTypeStr=boolean
  Out1 : Outport
  Out2 : Outport  Port=2
  wires:
  Logical Operator1/1 -> Out2/1
  In1/1 -> Half adder1/1(In1)
  Half adder2/1(Out1) -> Out1/1
  In2/1 -> Half adder1/2(In2)
  In3/1 -> Half adder2/2(In2)
  Half adder1/2(Out2) -> Logical Operator1/2
  Half adder1/1(Out1) -> Half adder2/1(In1)
  Half adder2/2(Out2) -> Logical Operator1/1

== system 8Bit_Processor/8-Bit_Processor/8-Bit_Multiplier/Full adder44 ==
  In1 : Inport  OutDataTypeStr=boolean
  In2 : Inport  Port=2  OutDataTypeStr=boolean
  In3 : Inport  Port=3  OutDataTypeStr=boolean
  Half adder1 : Subsystem
  Half adder2 : Subsystem
  Logical Operator1 : Logic  Operator=OR  AllPortsSameDT=off  OutDataTypeStr=boolean
  Out1 : Outport
  Out2 : Outport  Port=2
  wires:
  Logical Operator1/1 -> Out2/1
  In1/1 -> Half adder1/1(In1)
  Half adder2/1(Out1) -> Out1/1
  In2/1 -> Half adder1/2(In2)
  In3/1 -> Half adder2/2(In2)
  Half adder1/2(Out2) -> Logical Operator1/2
  Half adder1/1(Out1) -> Half adder2/1(In1)
  Half adder2/2(Out2) -> Logical Operator1/1

== system 8Bit_Processor/8-Bit_Processor/8-Bit_Multiplier/Full adder45 ==
  In1 : Inport  OutDataTypeStr=boolean
  In2 : Inport  Port=2  OutDataTypeStr=boolean
  In3 : Inport  Port=3  OutDataTypeStr=boolean
  Half adder1 : Subsystem
  Half adder2 : Subsystem
  Logical Operator1 : Logic  Operator=OR  AllPortsSameDT=off  OutDataTypeStr=boolean
  Out1 : Outport
  Out2 : Outport  Port=2
  wires:
  Logical Operator1/1 -> Out2/1
  In1/1 -> Half adder1/1(In1)
  Half adder2/1(Out1) -> Out1/1
  In2/1 -> Half adder1/2(In2)
  In3/1 -> Half adder2/2(In2)
  Half adder1/2(Out2) -> Logical Operator1/2
  Half adder1/1(Out1) -> Half adder2/1(In1)
  Half adder2/2(Out2) -> Logical Operator1/1

== system 8Bit_Processor/8-Bit_Processor/8-Bit_Multiplier/Full adder46 ==
  In1 : Inport  OutDataTypeStr=boolean
  In2 : Inport  Port=2  OutDataTypeStr=boolean
  In3 : Inport  Port=3  OutDataTypeStr=boolean
  Half adder1 : Subsystem
  Half adder2 : Subsystem
  Logical Operator1 : Logic  Operator=OR  AllPortsSameDT=off  OutDataTypeStr=boolean
  Out1 : Outport
  Out2 : Outport  Port=2
  wires:
  Logical Operator1/1 -> Out2/1
  In1/1 -> Half adder1/1(In1)
  Half adder2/1(Out1) -> Out1/1
  In2/1 -> Half adder1/2(In2)
  In3/1 -> Half adder2/2(In2)
  Half adder1/2(Out2) -> Logical Operator1/2
  Half adder1/1(Out1) -> Half adder2/1(In1)
  Half adder2/2(Out2) -> Logical Operator1/1

== system 8Bit_Processor/8-Bit_Processor/8-Bit_Multiplier/Full adder47 ==
  In1 : Inport  OutDataTypeStr=boolean
  In2 : Inport  Port=2  OutDataTypeStr=boolean
  In3 : Inport  Port=3  OutDataTypeStr=boolean
  Half adder1 : Subsystem
  Half adder2 : Subsystem
  Logical Operator1 : Logic  Operator=OR  AllPortsSameDT=off  OutDataTypeStr=boolean
  Out1 : Outport
  Out2 : Outport  Port=2
  wires:
  Logical Operator1/1 -> Out2/1
  In1/1 -> Half adder1/1(In1)
  Half adder2/1(Out1) -> Out1/1
  In2/1 -> Half adder1/2(In2)
  In3/1 -> Half adder2/2(In2)
  Half adder1/2(Out2) -> Logical Operator1/2
  Half adder1/1(Out1) -> Half adder2/1(In1)
  Half adder2/2(Out2) -> Logical Operator1/1

== system 8Bit_Processor/8-Bit_Processor/8-Bit_Multiplier/Full adder48 ==
  In1 : Inport  OutDataTypeStr=boolean
  In2 : Inport  Port=2  OutDataTypeStr=boolean
  In3 : Inport  Port=3  OutDataTypeStr=boolean
  Half adder1 : Subsystem
  Half adder2 : Subsystem
  Logical Operator1 : Logic  Operator=OR  AllPortsSameDT=off  OutDataTypeStr=boolean
  Out1 : Outport
  Out2 : Outport  Port=2
  wires:
  Logical Operator1/1 -> Out2/1
  In1/1 -> Half adder1/1(In1)
  Half adder2/1(Out1) -> Out1/1
  In2/1 -> Half adder1/2(In2)
  In3/1 -> Half adder2/2(In2)
  Half adder1/2(Out2) -> Logical Operator1/2
  Half adder1/1(Out1) -> Half adder2/1(In1)
  Half adder2/2(Out2) -> Logical Operator1/1

== system 8Bit_Processor/8-Bit_Processor/8-Bit_Multiplier/Full adder5 ==
  In1 : Inport  OutDataTypeStr=boolean
  In2 : Inport  Port=2  OutDataTypeStr=boolean
  In3 : Inport  Port=3  OutDataTypeStr=boolean
  Half adder1 : Subsystem
  Half adder2 : Subsystem
  Logical Operator1 : Logic  Operator=OR  AllPortsSameDT=off  OutDataTypeStr=boolean
  Out1 : Outport
  Out2 : Outport  Port=2
  wires:
  Logical Operator1/1 -> Out2/1
  In1/1 -> Half adder1/1(In1)
  Half adder2/1(Out1) -> Out1/1
  In2/1 -> Half adder1/2(In2)
  In3/1 -> Half adder2/2(In2)
  Half adder1/2(Out2) -> Logical Operator1/2
  Half adder1/1(Out1) -> Half adder2/1(In1)
  Half adder2/2(Out2) -> Logical Operator1/1

== system 8Bit_Processor/8-Bit_Processor/8-Bit_Multiplier/Full adder6 ==
  In1 : Inport  OutDataTypeStr=boolean
  In2 : Inport  Port=2  OutDataTypeStr=boolean
  In3 : Inport  Port=3  OutDataTypeStr=boolean
  Half adder1 : Subsystem
  Half adder2 : Subsystem
  Logical Operator1 : Logic  Operator=OR  AllPortsSameDT=off  OutDataTypeStr=boolean
  Out1 : Outport
  Out2 : Outport  Port=2
  wires:
  Logical Operator1/1 -> Out2/1
  In1/1 -> Half adder1/1(In1)
  Half adder2/1(Out1) -> Out1/1
  In2/1 -> Half adder1/2(In2)
  In3/1 -> Half adder2/2(In2)
  Half adder1/2(Out2) -> Logical Operator1/2
  Half adder1/1(Out1) -> Half adder2/1(In1)
  Half adder2/2(Out2) -> Logical Operator1/1

== system 8Bit_Processor/8-Bit_Processor/8-Bit_Multiplier/Full adder7 ==
  In1 : Inport  OutDataTypeStr=boolean
  In2 : Inport  Port=2  OutDataTypeStr=boolean
  In3 : Inport  Port=3  OutDataTypeStr=boolean
  Half adder1 : Subsystem
  Half adder2 : Subsystem
  Logical Operator1 : Logic  Operator=OR  AllPortsSameDT=off  OutDataTypeStr=boolean
  Out1 : Outport
  Out2 : Outport  Port=2
  wires:
  Logical Operator1/1 -> Out2/1
  In1/1 -> Half adder1/1(In1)
  Half adder2/1(Out1) -> Out1/1
  In2/1 -> Half adder1/2(In2)
  In3/1 -> Half adder2/2(In2)
  Half adder1/2(Out2) -> Logical Operator1/2
  Half adder1/1(Out1) -> Half adder2/1(In1)
  Half adder2/2(Out2) -> Logical Operator1/1

== system 8Bit_Processor/8-Bit_Processor/8-Bit_Multiplier/Full adder8 ==
  In1 : Inport  OutDataTypeStr=boolean
  In2 : Inport  Port=2  OutDataTypeStr=boolean
  In3 : Inport  Port=3  OutDataTypeStr=boolean
  Half adder1 : Subsystem
  Half adder2 : Subsystem
  Logical Operator1 : Logic  Operator=OR  AllPortsSameDT=off  OutDataTypeStr=boolean
  Out1 : Outport
  Out2 : Outport  Port=2
  wires:
  Logical Operator1/1 -> Out2/1
  In1/1 -> Half adder1/1(In1)
  Half adder2/1(Out1) -> Out1/1
  In2/1 -> Half adder1/2(In2)
  In3/1 -> Half adder2/2(In2)
  Half adder1/2(Out2) -> Logical Operator1/2
  Half adder1/1(Out1) -> Half adder2/1(In1)
  Half adder2/2(Out2) -> Logical Operator1/1

== system 8Bit_Processor/8-Bit_Processor/8-Bit_Multiplier/Full adder9 ==
  In1 : Inport  OutDataTypeStr=boolean
  In2 : Inport  Port=2  OutDataTypeStr=boolean
  In3 : Inport  Port=3  OutDataTypeStr=boolean
  Half adder1 : Subsystem
  Half adder2 : Subsystem
  Logical Operator1 : Logic  Operator=OR  AllPortsSameDT=off  OutDataTypeStr=boolean
  Out1 : Outport
  Out2 : Outport  Port=2
  wires:
  Logical Operator1/1 -> Out2/1
  In1/1 -> Half adder1/1(In1)
  Half adder2/1(Out1) -> Out1/1
  In2/1 -> Half adder1/2(In2)
  In3/1 -> Half adder2/2(In2)
  Half adder1/2(Out2) -> Logical Operator1/2
  Half adder1/1(Out1) -> Half adder2/1(In1)
  Half adder2/2(Out2) -> Logical Operator1/1

== system 8Bit_Processor/8-Bit_Processor/8-Bit_Multiplier/Half adder1 ==
  In1 : Inport  OutDataTypeStr=boolean
  In2 : Inport  Port=2  OutDataTypeStr=boolean
  Logical Operator : Logic  AllPortsSameDT=off  OutDataTypeStr=boolean
  Logical Operator1 : Logic  Operator=XOR  AllPortsSameDT=off  OutDataTypeStr=boolean
  Out1 : Outport
  Out2 : Outport  Port=2
  wires:
  In2/1 -> Logical Operator/2, Logical Operator1/2
  In1/1 -> Logical Operator/1, Logical Operator1/1
  Logical Operator1/1 -> Out1/1
  Logical Operator/1 -> Out2/1

== system 8Bit_Processor/8-Bit_Processor/8-Bit_Multiplier/Half adder2 ==
  In1 : Inport  OutDataTypeStr=boolean
  In2 : Inport  Port=2  OutDataTypeStr=boolean
  Logical Operator : Logic  AllPortsSameDT=off  OutDataTypeStr=boolean
  Logical Operator1 : Logic  Operator=XOR  AllPortsSameDT=off  OutDataTypeStr=boolean
  Out1 : Outport
  Out2 : Outport  Port=2
  wires:
  In2/1 -> Logical Operator/2, Logical Operator1/2
  In1/1 -> Logical Operator/1, Logical Operator1/1
  Logical Operator1/1 -> Out1/1
  Logical Operator/1 -> Out2/1

== system 8Bit_Processor/8-Bit_Processor/8-Bit_Multiplier/Half adder3 ==
  In1 : Inport  OutDataTypeStr=boolean
  In2 : Inport  Port=2  OutDataTypeStr=boolean
  Logical Operator : Logic  AllPortsSameDT=off  OutDataTypeStr=boolean
  Logical Operator1 : Logic  Operator=XOR  AllPortsSameDT=off  OutDataTypeStr=boolean
  Out1 : Outport
  Out2 : Outport  Port=2
  wires:
  In2/1 -> Logical Operator/2, Logical Operator1/2
  In1/1 -> Logical Operator/1, Logical Operator1/1
  Logical Operator1/1 -> Out1/1
  Logical Operator/1 -> Out2/1

== system 8Bit_Processor/8-Bit_Processor/8-Bit_Multiplier/Half adder4 ==
  In1 : Inport  OutDataTypeStr=boolean
  In2 : Inport  Port=2  OutDataTypeStr=boolean
  Logical Operator : Logic  AllPortsSameDT=off  OutDataTypeStr=boolean
  Logical Operator1 : Logic  Operator=XOR  AllPortsSameDT=off  OutDataTypeStr=boolean
  Out1 : Outport
  Out2 : Outport  Port=2
  wires:
  In2/1 -> Logical Operator/2, Logical Operator1/2
  In1/1 -> Logical Operator/1, Logical Operator1/1
  Logical Operator1/1 -> Out1/1
  Logical Operator/1 -> Out2/1

== system 8Bit_Processor/8-Bit_Processor/8-Bit_Multiplier/Half adder5 ==
  In1 : Inport  OutDataTypeStr=boolean
  In2 : Inport  Port=2  OutDataTypeStr=boolean
  Logical Operator : Logic  AllPortsSameDT=off  OutDataTypeStr=boolean
  Logical Operator1 : Logic  Operator=XOR  AllPortsSameDT=off  OutDataTypeStr=boolean
  Out1 : Outport
  Out2 : Outport  Port=2
  wires:
  In2/1 -> Logical Operator/2, Logical Operator1/2
  In1/1 -> Logical Operator/1, Logical Operator1/1
  Logical Operator1/1 -> Out1/1
  Logical Operator/1 -> Out2/1

== system 8Bit_Processor/8-Bit_Processor/8-Bit_Multiplier/Half adder6 ==
  In1 : Inport  OutDataTypeStr=boolean
  In2 : Inport  Port=2  OutDataTypeStr=boolean
  Logical Operator : Logic  AllPortsSameDT=off  OutDataTypeStr=boolean
  Logical Operator1 : Logic  Operator=XOR  AllPortsSameDT=off  OutDataTypeStr=boolean
  Out1 : Outport
  Out2 : Outport  Port=2
  wires:
  In2/1 -> Logical Operator/2, Logical Operator1/2
  In1/1 -> Logical Operator/1, Logical Operator1/1
  Logical Operator1/1 -> Out1/1
  Logical Operator/1 -> Out2/1

== system 8Bit_Processor/8-Bit_Processor/8-Bit_Multiplier/Half adder7 ==
  In1 : Inport  OutDataTypeStr=boolean
  In2 : Inport  Port=2  OutDataTypeStr=boolean
  Logical Operator : Logic  AllPortsSameDT=off  OutDataTypeStr=boolean
  Logical Operator1 : Logic  Operator=XOR  AllPortsSameDT=off  OutDataTypeStr=boolean
  Out1 : Outport
  Out2 : Outport  Port=2
  wires:
  In2/1 -> Logical Operator/2, Logical Operator1/2
  In1/1 -> Logical Operator/1, Logical Operator1/1
  Logical Operator1/1 -> Out1/1
  Logical Operator/1 -> Out2/1

== system 8Bit_Processor/8-Bit_Processor/8-Bit_Multiplier/Half adder8 ==
  In1 : Inport  OutDataTypeStr=boolean
  In2 : Inport  Port=2  OutDataTypeStr=boolean
  Logical Operator : Logic  AllPortsSameDT=off  OutDataTypeStr=boolean
  Logical Operator1 : Logic  Operator=XOR  AllPortsSameDT=off  OutDataTypeStr=boolean
  Out1 : Outport
  Out2 : Outport  Port=2
  wires:
  In2/1 -> Logical Operator/2, Logical Operator1/2
  In1/1 -> Logical Operator/1, Logical Operator1/1
  Logical Operator1/1 -> Out1/1
  Logical Operator/1 -> Out2/1

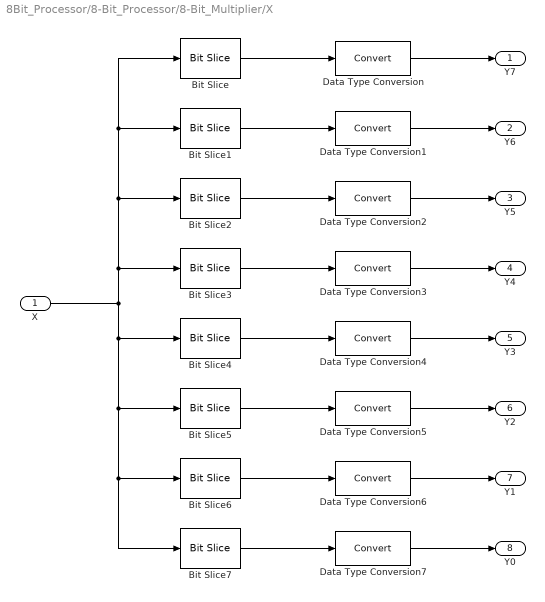
== system 8Bit_Processor/8-Bit_Processor/8-Bit_Multiplier/X ==
  X : Inport  OutDataTypeStr=uint8  SampleTime=1
  Bit Slice : hdlsllib/Logic and Bit Operations/Bit Slice  lidx=7  ridx=7
      settings: SourceProductName=Simulink  SourceProductBaseCode=SL
  Bit Slice1 : hdlsllib/Logic and Bit Operations/Bit Slice  lidx=6  ridx=6
      settings: SourceProductName=Simulink  SourceProductBaseCode=SL
  Bit Slice2 : hdlsllib/Logic and Bit Operations/Bit Slice  lidx=5  ridx=5
      settings: SourceProductName=Simulink  SourceProductBaseCode=SL
  Bit Slice3 : hdlsllib/Logic and Bit Operations/Bit Slice  lidx=4  ridx=4
      settings: SourceProductName=Simulink  SourceProductBaseCode=SL
  Bit Slice4 : hdlsllib/Logic and Bit Operations/Bit Slice  lidx=3  ridx=3
      settings: SourceProductName=Simulink  SourceProductBaseCode=SL
  Bit Slice5 : hdlsllib/Logic and Bit Operations/Bit Slice  lidx=2  ridx=2
      settings: SourceProductName=Simulink  SourceProductBaseCode=SL
  Bit Slice6 : hdlsllib/Logic and Bit Operations/Bit Slice  lidx=1  ridx=1
      settings: SourceProductName=Simulink  SourceProductBaseCode=SL
  Bit Slice7 : hdlsllib/Logic and Bit Operations/Bit Slice  lidx=0  ridx=0
      settings: SourceProductName=Simulink  SourceProductBaseCode=SL
  Data Type Conversion{,1..7} (8 alike) : DataTypeConversion
  Y7 : Outport
  Y6 : Outport  Port=2
  Y5 : Outport  Port=3
  Y4 : Outport  Port=4
  Y3 : Outport  Port=5
  Y2 : Outport  Port=6
  Y1 : Outport  Port=7
  Y0 : Outport  Port=8
  wires:
  Bit Slice6/1 -> Data Type Conversion6/1
  X/1 -> Bit Slice3/1, Bit Slice2/1, Bit Slice1/1, Bit Slice/1, Bit Slice4/1, Bit Slice5/1, Bit Slice6/1, Bit Slice7/1
  Bit Slice/1 -> Data Type Conversion/1
  Bit Slice7/1 -> Data Type Conversion7/1
  Bit Slice4/1 -> Data Type Conversion4/1
  Bit Slice1/1 -> Data Type Conversion1/1
  Bit Slice3/1 -> Data Type Conversion3/1
  Data Type Conversion1/1 -> Y6/1
  Data Type Conversion7/1 -> Y0/1
  Data Type Conversion5/1 -> Y2/1
  Data Type Conversion3/1 -> Y4/1
  Data Type Conversion4/1 -> Y3/1
  Bit Slice2/1 -> Data Type Conversion2/1
  Bit Slice5/1 -> Data Type Conversion5/1
  Data Type Conversion6/1 -> Y1/1
  Data Type Conversion/1 -> Y7/1
  Data Type Conversion2/1 -> Y5/1
